simulink model "TP3Gravity"  (R2017b)
settings: Solver=VariableStepAuto  StartTime=0.0  StopTime=10.0  RelTol=1e-3
values from neighbouring files (symbols this model uses):
  dt = 0.001    [TP3Au422_Main.m]    (also in TP3Combined_Main.m; TP3DC_Main.m; TP3Q3_Main.m)
  F_dis1 = 150    [TP3Au422_Main.m]    (also in TP3Combined_Main.m = 0; TP3DC_Main.m; TP3Q3_Main.m = 0)
  F_dis2 = -107.5    [TP3Au422_Main.m]    (also in TP3Combined_Main.m = 0; TP3DC_Main.m; TP3Q3_Main.m = 0)
  Kd = 5    [TP3Au422_Main.m]    (also in TP3Combined_Main.m = 3; TP3DC_Main.m = 3; TP3Q3_Main.m = 3)
  Kp = 50    [TP3Au422_Main.m]    (also in TP3Combined_Main.m = 6; TP3DC_Main.m = 6; TP3Q3_Main.m = 6)
  m = 1    [TP3Au422_Main.m]    (also in TP3Combined_Main.m; TP3DC_Main.m; TP3Q3_Main.m)
  t_dis1 = 20    [TP3Au422_Main.m]    (also in TP3Combined_Main.m; TP3DC_Main.m; TP3Q3_Main.m)
  t_dis2 = 40    [TP3Au422_Main.m]    (also in TP3Combined_Main.m; TP3DC_Main.m; TP3Q3_Main.m)
  Variance = 0.75    [TP3Au422_Main.m]
undefined symbols (not defined in the file or in its folder): xd
libraries: dspsrcs4 x3
settings Model: Creator=Huynh  LastModifiedBy=Huynh

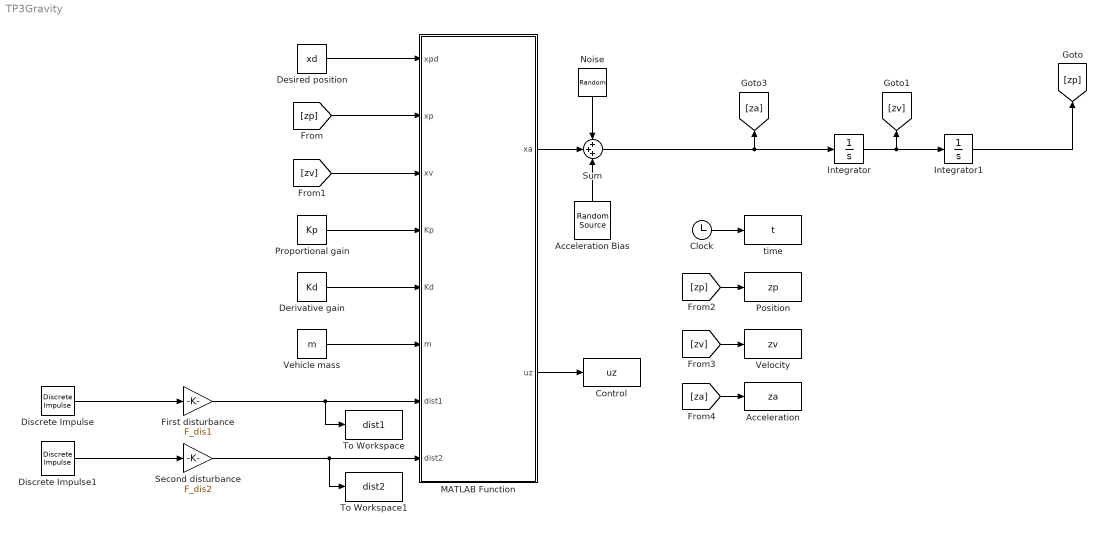
== system TP3Gravity ==
  Acceleration : ToWorkspace  VariableName=za  SampleTime=dt
  Acceleration Bias : dspsrcs4/Random Source  SrcType=Uniform  NormMethod=Ziggurat  CltLength=12  MinVal=Min  MaxVal=Max  MeanVal=0  VarVal=1  RepMode=Not repeatable  rawSeed=1  IsInherit=off  SampMode=Discrete  SampTime=Bias_Sample_time  SampFrame=1  DataType=Double  OutComplex=Real  OutputFrames=off
  Clock : Clock
  Control : ToWorkspace  VariableName=uz  SampleTime=dt
  Derivative gain : Constant  Value=Kd
  Desired position : Constant  Value=xd
  Discrete Impulse : dspsrcs4/Discrete  Impulse  Delay=t_dis1/dt  SampleTime=dt  FrameSample=1  OutputFrames=off  dataType=double  isSigned=on  wordLen=16  udDataType=sfix(16)  fracBitsMode=Best precision  numFracBits=15  OutDataTypeStr=double  LastOutDataTypeStr=double
  Discrete Impulse1 : dspsrcs4/Discrete  Impulse  Delay=t_dis2/dt  SampleTime=dt  FrameSample=1  OutputFrames=off  dataType=double  isSigned=on  wordLen=16  udDataType=sfix(16)  fracBitsMode=Best precision  numFracBits=15  OutDataTypeStr=double  LastOutDataTypeStr=double
  First disturbance : Gain  Gain=F_dis1
  Integrator : Integrator
  Integrator1 : Integrator
  MATLAB Function : MATLAB Function  TreatAsAtomicUnit=on
  Noise : RandomNumber  Variance=Variance  SampleTime=dt
  Position : ToWorkspace  VariableName=zp  SampleTime=dt
  Proportional gain : Constant  Value=Kp
  Second disturbance : Gain  Gain=F_dis2
  Sum : Sum  Inputs=+++
  To Workspace : ToWorkspace  VariableName=dist1  SampleTime=dt
      settings: Save2DSignal=2-D array (concatenate along first dimension)
  To Workspace1 : ToWorkspace  VariableName=dist2  SampleTime=dt
      settings: Save2DSignal=2-D array (concatenate along first dimension)
  Vehicle mass : Constant  Value=m
  Velocity : ToWorkspace  VariableName=zv  SampleTime=dt
  time : ToWorkspace  VariableName=t  SampleTime=dt
  wires:
  [zv] -> MATLAB Function/3(xv)
  Vehicle mass/1 -> MATLAB Function/6(m)
  Clock/1 -> time/1
  Derivative gain/1 -> MATLAB Function/5(Kd)
  Discrete Impulse/1 -> First disturbance/1
  [zv] -> Velocity/1
  Discrete Impulse1/1 -> Second disturbance/1
  Sum/1 -> [za], Integrator/1
  MATLAB Function/1(xa) -> Sum/2
  Integrator/1 -> [zv], Integrator1/1
  Noise/1 -> Sum/1
  First disturbance/1 -> To Workspace/1, MATLAB Function/7(dist1)
  Second disturbance/1 -> To Workspace1/1, MATLAB Function/8(dist2)
  [za] -> Acceleration/1
  MATLAB Function/2(uz) -> Control/1
  Desired position/1 -> MATLAB Function/1(xpd)
  Integrator1/1 -> [zp]
  [zp] -> Position/1
  Proportional gain/1 -> MATLAB Function/4(Kp)
  [zp] -> MATLAB Function/2(xp)
  Acceleration Bias/1 -> Sum/3

== matlab function TP3Gravity/MATLAB Function ==
  data: xpd input; xa output; xp input; xv input; Kp input; Kd input; m input; dist1 input; dist2 input; uz output
function [xa, uz] = PD(xpd, xp, xv, Kp, Kd, m, dist1, dist2) %PD Function

exp = xpd - xp; %Position error
exv = 0 - xv; %Velocity error

U = m * 9.81 * xp;%Potential energy
g = m * 9.81 ;
uz = Kp * exp + Kd * exv + g; %Control law equation
if uz > 20
    uz = 20;
elseif uz < -10
    uz = -10;
end
xa = (uz + dist1 + dist2 - 9.81 * m) / m ; %Acceleration update with disturbances
